simulink model "assignment4"  (R2017b)
settings: Solver=VariableStepAuto  StartTime=0.0  StopTime=10.0  RelTol=1e-3
settings Model: Creator=Raymond  LastModifiedBy=Raymond

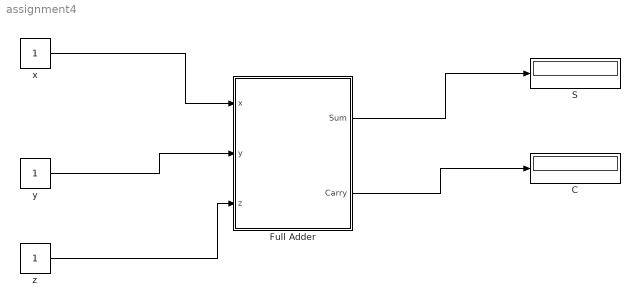
== system assignment4 ==
  C : Display
  Full Adder : Subsystem
  S : Display
  x : Constant  OutDataTypeStr=boolean
  y : Constant  OutDataTypeStr=boolean
  z : Constant  OutDataTypeStr=boolean
  wires:
  x/1 -> Full Adder/1(x)
  y/1 -> Full Adder/2(y)
  z/1 -> Full Adder/3(z)
  Full Adder/1(Sum) -> S/1
  Full Adder/2(Carry) -> C/1

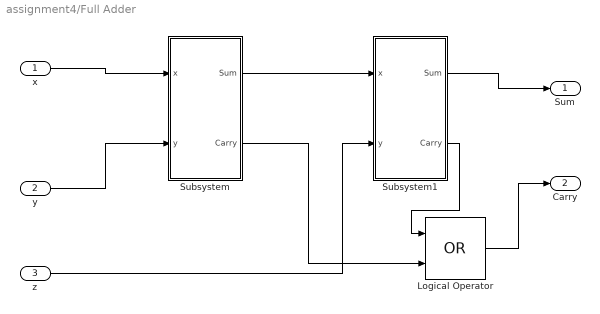
== system assignment4/Full Adder ==
  x : Inport
  y : Inport  Port=2
  z : Inport  Port=3
  Logical Operator : Logic  Operator=OR  IconShape=distinctive  AllPortsSameDT=off  OutDataTypeStr=boolean
  Subsystem : Subsystem
  Subsystem1 : Subsystem
  Sum : Outport
  Carry : Outport  Port=2
  wires:
  z/1 -> Subsystem1/2(y)
  Subsystem/2(Carry) -> Logical Operator/2
  Subsystem1/1(Sum) -> Sum/1
  x/1 -> Subsystem/1(x)
  y/1 -> Subsystem/2(y)
  Subsystem/1(Sum) -> Subsystem1/1(x)
  Subsystem1/2(Carry) -> Logical Operator/1
  Logical Operator/1 -> Carry/1

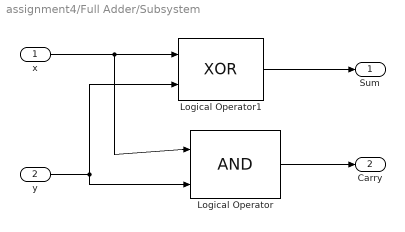
== system assignment4/Full Adder/Subsystem ==
  x : Inport
  y : Inport  Port=2
  Logical Operator : Logic  IconShape=distinctive  AllPortsSameDT=off  OutDataTypeStr=boolean
  Logical Operator1 : Logic  Operator=XOR  IconShape=distinctive  AllPortsSameDT=off  OutDataTypeStr=boolean
  Sum : Outport
  Carry : Outport  Port=2
  wires:
  x/1 -> Logical Operator/1, Logical Operator1/1
  y/1 -> Logical Operator1/2, Logical Operator/2
  Logical Operator/1 -> Carry/1
  Logical Operator1/1 -> Sum/1

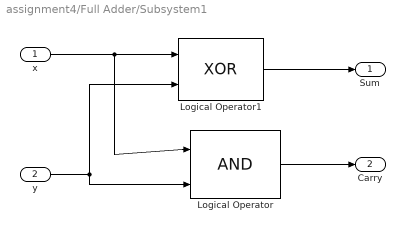
== system assignment4/Full Adder/Subsystem1 ==
  x : Inport
  y : Inport  Port=2
  Logical Operator : Logic  IconShape=distinctive  AllPortsSameDT=off  OutDataTypeStr=boolean
  Logical Operator1 : Logic  Operator=XOR  IconShape=distinctive  AllPortsSameDT=off  OutDataTypeStr=boolean
  Sum : Outport
  Carry : Outport  Port=2
  wires:
  x/1 -> Logical Operator/1, Logical Operator1/1
  y/1 -> Logical Operator1/2, Logical Operator/2
  Logical Operator/1 -> Carry/1
  Logical Operator1/1 -> Sum/1
